simulink model "Demo"  (R2020b)
settings: Solver=FixedStepAuto  StartTime=0.0  StopTime=10.0  RelTol=1e-3
settings Model: Creator=AG77579  LastModifiedBy=AG77579

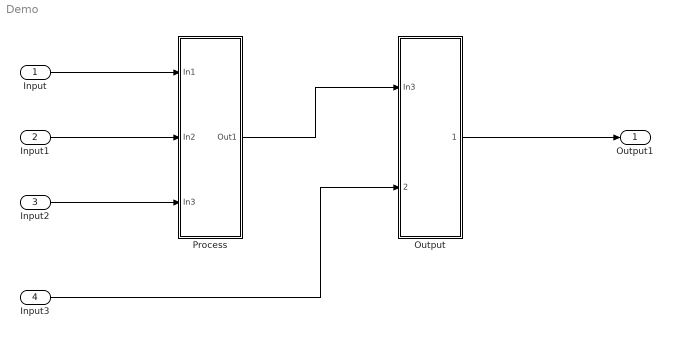
== system Demo ==
  Input : Inport
  Input1 : Inport  Port=2
  Input2 : Inport  Port=3
  Input3 : Inport  Port=4
  Output : Subsystem
  Process : Subsystem
  Output1 : Outport
  wires:
  Input/1 -> Process/1(In1)
  Input1/1 -> Process/2(In2)
  Input2/1 -> Process/3(In3)
  Process/1(Out1) -> Output/1(In3)
  Input3/1 -> Output/2(Input3)
  Output/1(Output1) -> Output1/1

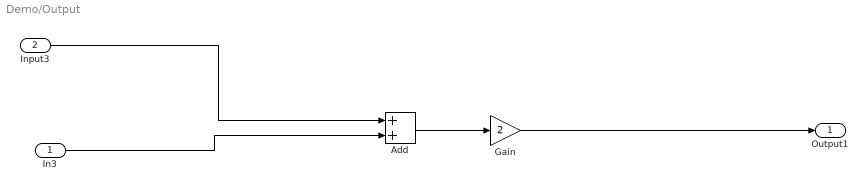
== system Demo/Output ==
  In3 : Inport
  Input3 : Inport  Port=2
  Add : Sum
  Gain : Gain  Gain=2
  Output1 : Outport
  wires:
  Input3/1 -> Add/1
  In3/1 -> Add/2
  Add/1 -> Gain/1
  Gain/1 -> Output1/1

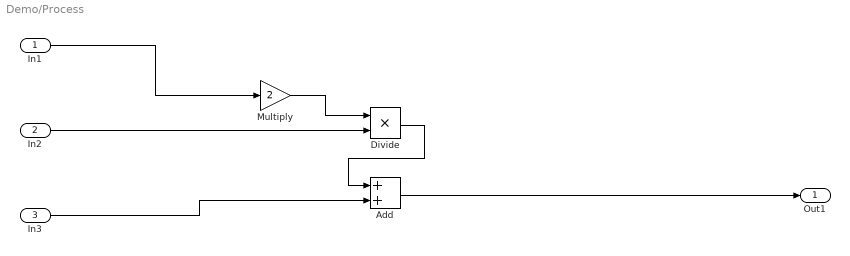
== system Demo/Process ==
  In1 : Inport
  In2 : Inport  Port=2
  In3 : Inport  Port=3
  Add : Sum
  Divide : Product  Inputs=**
  Multiply : Gain  Gain=2
  Out1 : Outport
  wires:
  Multiply/1 -> Divide/1
  In2/1 -> Divide/2
  Add/1 -> Out1/1
  In3/1 -> Add/2
  Divide/1 -> Add/1
  In1/1 -> Multiply/1
